simulink model "Tactical_SC_traincgf_4_15_Nov_27_Block"  (R2021a)
settings: Solver=VariableStepAuto  StartTime=0.0  StopTime=10.0  RelTol=1e-3
libraries: neural x66
(part 3 of 3)

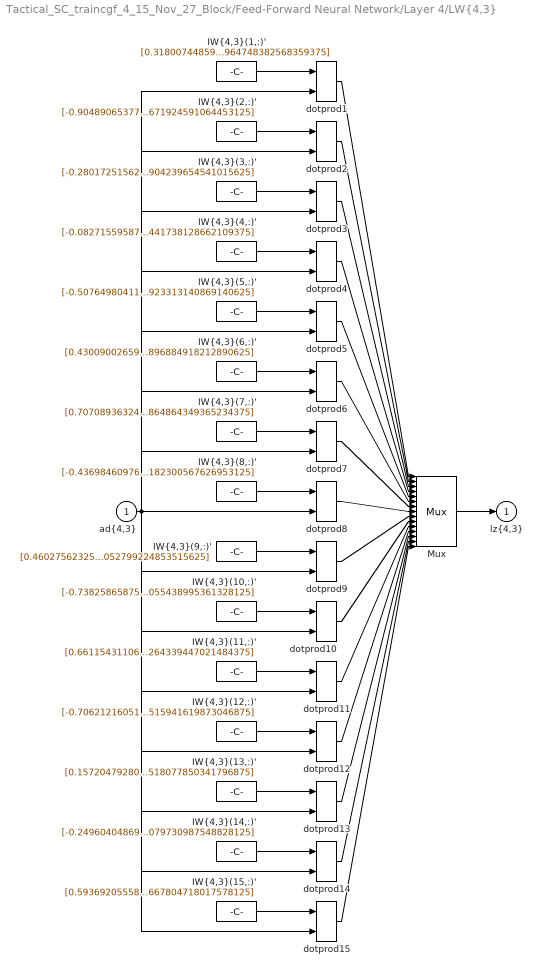
== system Tactical_SC_traincgf_4_15_Nov_27_Block/Feed-Forward Neural Network/Layer 4/LW{4,3} ==
  "ad{4,3}" : Inport  PortDimensions=15
      mask Display: e = 0.06;c1 = [120 230 180]/255;c2 = ([120 230 180]+0)/(256+128);c3 = ([120 230 180]+128)/(256+128);patch([0 1 1 0],[0 0 1 1],c1);patch([0 1 1 1-e 1-e 0+e],[0 0 1 1-e 0+e 0+e],c2);patch([0 0 1 1-e 0+e 0+e],[0 1 1 1-e 1-e 0+e],c3);plot([0 1 1 0 0],[0 0 1 1 0]);
  "IW{4,3}(1,:)'" : Constant  Value=[0.318007448593325692254296654937206767499446868896484375;0.0075615715523118520735579295433126389980316162109375;-0.96361569277834124847004204639233648777008056640625;0.860487806043781500164868702995590865612030029296875;0.7524752577316433654885940995882265269756317138671875;0.0077755469209772609673336773994378745555877685546875;-0.422356185153830387957185621417011134326457977294921875;0.6601121326122356691712411702610552310943603515625;0.510717921416298015202528404188342392444610595703125;-0.1037827559143178479672542380285449326038360595703125;-0.21994697437200461109796378877945244312286376953125;-0.7659263609886843848784110377891920506954193115234375;0.6680132640011307021410402740002609789371490478515625;0.99866317249397440480862542244722135365009307861328125;0.86246253723063259766234978087595663964748382568359375]
      mask Display: e = 0.06;c1 = [120 150 230]/255;c2 = ([120 150 230]+0)/383;c3 = ([120 150 230]+128)/383;patch([0 1 1 0],[0 0 1 1],c1);patch([0 1 1 1-e 1-e 0+e],[0 0 1 1-e 0+e 0+e],c2);patch([0 0 1 1-e 0+e 0+e],[0 1 1 1-e 1-e 0+e],c3);plot([0 1 1 0 0],[0 0 1 1 0]);disp('weights');
  "IW{4,3}(10,:)'" : Constant  Value=[-0.73825865875039620167541443152003921568393707275390625;0.334240600080149885542368792812339961528778076171875;-0.34759286482494566872247787614469416439533233642578125;-0.8904164201605351269819266235572285950183868408203125;0.6651335768264690084805579317617230117321014404296875;-0.732992280677375429576159149291925132274627685546875;-0.932434493180203549655971073661930859088897705078125;-0.85344556112142255788199918242753483355045318603515625;0.73189389910298052743797825314686633646488189697265625;-0.2192027742775237986183611837986973114311695098876953125;0.7688100905519898997653172045829705893993377685546875;-0.2037382409373282854403441888280212879180908203125;-0.803239734476193678602840009261853992938995361328125;-0.1369989655326274424762544867917313240468502044677734375;-0.59536079412170039848462010922958143055438995361328125]
      mask Display: e = 0.06;c1 = [120 150 230]/255;c2 = ([120 150 230]+0)/383;c3 = ([120 150 230]+128)/383;patch([0 1 1 0],[0 0 1 1],c1);patch([0 1 1 1-e 1-e 0+e],[0 0 1 1-e 0+e 0+e],c2);patch([0 0 1 1-e 0+e 0+e],[0 1 1 1-e 1-e 0+e],c3);plot([0 1 1 0 0],[0 0 1 1 0]);disp('weights');
  "IW{4,3}(11,:)'" : Constant  Value=[0.6611543110624340524594799717306159436702728271484375;0.172879229357835839664403465576469898223876953125;-0.73239400543458577086397554012364707887172698974609375;-0.388976697640453117355008316735620610415935516357421875;-0.1647486253821566493105166273380746133625507354736328125;-0.9568882255930060143356286062044091522693634033203125;-0.08967440119208837379094489961062208749353885650634765625;-0.1867190373629059318982825743660214357078075408935546875;0.74064277100053121927203392260707914829254150390625;-0.53590128485240129396771635583718307316303253173828125;0.4417113416338629416912908709491603076457977294921875;0.03073443842314471652343854657374322414398193359375;-0.67744238093146780244069304899312555789947509765625;0.69070075771987549106967207990237511694431304931640625;-0.090605605861847793303098796968697570264339447021484375]
      mask Display: e = 0.06;c1 = [120 150 230]/255;c2 = ([120 150 230]+0)/383;c3 = ([120 150 230]+128)/383;patch([0 1 1 0],[0 0 1 1],c1);patch([0 1 1 1-e 1-e 0+e],[0 0 1 1-e 0+e 0+e],c2);patch([0 0 1 1-e 0+e 0+e],[0 1 1 1-e 1-e 0+e],c3);plot([0 1 1 0 0],[0 0 1 1 0]);disp('weights');
  "IW{4,3}(12,:)'" : Constant  Value=[-0.7062121605125781798051320947706699371337890625;0.3502248328102306462739079506718553602695465087890625;-0.29514974520824022174991796418908052146434783935546875;-0.910971163136844896968113971524871885776519775390625;-0.04374406409938964845895981170542654581367969512939453125;0.11968141174501933932106112479232251644134521484375;0.264553137550485095719210448805824853479862213134765625;0.331907915136774145370424093925976194441318511962890625;0.126991008466725119330220650226692669093608856201171875;0.451463364557955715294923493274836800992488861083984375;-0.9627744505472277669611003148020245134830474853515625;0.315061084191821993982784988475032150745391845703125;0.2361511563990832396342511856346391141414642333984375;-0.2392189610648267628079111091210506856441497802734375;-0.146865284912714055831628456871840171515941619873046875]
      mask Display: e = 0.06;c1 = [120 150 230]/255;c2 = ([120 150 230]+0)/383;c3 = ([120 150 230]+128)/383;patch([0 1 1 0],[0 0 1 1],c1);patch([0 1 1 1-e 1-e 0+e],[0 0 1 1-e 0+e 0+e],c2);patch([0 0 1 1-e 0+e 0+e],[0 1 1 1-e 1-e 0+e],c3);plot([0 1 1 0 0],[0 0 1 1 0]);disp('weights');
  "IW{4,3}(13,:)'" : Constant  Value=[0.1572047928025288310305285222057136707007884979248046875;-0.2779559016106782909361072597675956785678863525390625;-0.7640312274407909942652850077138282358646392822265625;-0.604037151232293734182121625053696334362030029296875;0.1039704250373072458302203813218511641025543212890625;-0.3983619638610218505192506199819035828113555908203125;0.06345107524350544758728887018150999210774898529052734375;0.8674513190918593519285195725387893617153167724609375;0.166115950281934543486528355060727335512638092041015625;-0.46473978853246522557896014404832385480403900146484375;0.3495529342565715236190726500353775918483734130859375;0.9018303965299183655446313423453830182552337646484375;0.7396095696434386024264995285193435847759246826171875;0.27563280297923220540923239241237752139568328857421875;0.92522961385834878722533858308452181518077850341796875]
      mask Display: e = 0.06;c1 = [120 150 230]/255;c2 = ([120 150 230]+0)/383;c3 = ([120 150 230]+128)/383;patch([0 1 1 0],[0 0 1 1],c1);patch([0 1 1 1-e 1-e 0+e],[0 0 1 1-e 0+e 0+e],c2);patch([0 0 1 1-e 0+e 0+e],[0 1 1 1-e 1-e 0+e],c3);plot([0 1 1 0 0],[0 0 1 1 0]);disp('weights');
  "IW{4,3}(14,:)'" : Constant  Value=[-0.2496040486909129330062029339387663640081882476806640625;0.24055685414217098383460324839688837528228759765625;0.77732094229939596718992333990172483026981353759765625;0.436514146718682827241764243808574974536895751953125;-0.445911323119876523701776704911026172339916229248046875;0.878819427746916570498569853953085839748382568359375;-0.285655534964172563849871266938862390816211700439453125;0.620303798530214667295012986869551241397857666015625;-0.69046142052182946091676285504945553839206695556640625;0.81167656367563367769690785280545242130756378173828125;-0.1229823515269743428035553733934648334980010986328125;0.444697028654995829555218733730725944042205810546875;0.9206352224126470584764092564000748097896575927734375;0.60650102629068836090908689584466628730297088623046875;0.2377285168034162510242168764307280071079730987548828125]
      mask Display: e = 0.06;c1 = [120 150 230]/255;c2 = ([120 150 230]+0)/383;c3 = ([120 150 230]+128)/383;patch([0 1 1 0],[0 0 1 1],c1);patch([0 1 1 1-e 1-e 0+e],[0 0 1 1-e 0+e 0+e],c2);patch([0 0 1 1-e 0+e 0+e],[0 1 1 1-e 1-e 0+e],c3);plot([0 1 1 0 0],[0 0 1 1 0]);disp('weights');
  "IW{4,3}(15,:)'" : Constant  Value=[0.59369205558419835266903419324080459773540496826171875;0.6223017702005704254730744651169516146183013916015625;-0.82303653443154389801605930188088677823543548583984375;0.447647643950220885944446536086616106331348419189453125;0.478950635277783864918177414438105188310146331787109375;0.961807272093718079730706449481658637523651123046875;0.907417665800277717380595277063548564910888671875;-0.0279287499802652085245657787027084850706160068511962890625;0.78449887606904689096865013198112137615680694580078125;0.6276639944286017680497025139629840850830078125;-0.1243596416674599414164958943729288876056671142578125;-0.1998405092753248180059699734556488692760467529296875;0.173164233800528755136127756486530415713787078857421875;0.80725476240327120880380107337259687483310699462890625;0.394073676563273966877432030742056667804718017578125]
      mask Display: e = 0.06;c1 = [120 150 230]/255;c2 = ([120 150 230]+0)/383;c3 = ([120 150 230]+128)/383;patch([0 1 1 0],[0 0 1 1],c1);patch([0 1 1 1-e 1-e 0+e],[0 0 1 1-e 0+e 0+e],c2);patch([0 0 1 1-e 0+e 0+e],[0 1 1 1-e 1-e 0+e],c3);plot([0 1 1 0 0],[0 0 1 1 0]);disp('weights');
  "IW{4,3}(2,:)'" : Constant  Value=[-0.904890653772267850030175395659171044826507568359375;-0.0208113225532915446791548674809746444225311279296875;-0.8322529834342002885705369408242404460906982421875;-0.201960061930889001047262354404665529727935791015625;0.1648659289748206635550786813837476074695587158203125;0.293619332545560940417317397077567875385284423828125;0.601640573903069242334140653838403522968292236328125;0.698170959908910315760977027821354568004608154296875;-0.1659050925144660570964560974971391260623931884765625;-0.5886553210720730788807486533187329769134521484375;-0.004194114071626842132900492288172245025634765625;0.629363379037164438756235540495254099369049072265625;-0.7313233165425836457274044732912443578243255615234375;0.1070831469910651367882792328600771725177764892578125;-0.61843070398175559176934257266111671924591064453125]
      mask Display: e = 0.06;c1 = [120 150 230]/255;c2 = ([120 150 230]+0)/383;c3 = ([120 150 230]+128)/383;patch([0 1 1 0],[0 0 1 1],c1);patch([0 1 1 1-e 1-e 0+e],[0 0 1 1-e 0+e 0+e],c2);patch([0 0 1 1-e 0+e 0+e],[0 1 1 1-e 1-e 0+e],c3);plot([0 1 1 0 0],[0 0 1 1 0]);disp('weights');
  "IW{4,3}(3,:)'" : Constant  Value=[-0.2801725156256142934552144652116112411022186279296875;0.754097446770087831424689284176565706729888916015625;0.9614352930014380405054907896555960178375244140625;-0.89902945368803965919823895092122256755828857421875;-0.83854787826719501264705058929393999278545379638671875;-0.384508835938118576081024002633057534694671630859375;0.78776955048410834958616533185704611241817474365234375;-0.25780397740523997018868840314098633825778961181640625;0.984262714168782082424513646401464939117431640625;0.8275349590010059319666879673604853451251983642578125;0.389610385344987708577946250443346798419952392578125;-0.3502891227389819395199310747557319700717926025390625;-0.8684364926597070155622759557445533573627471923828125;0.040764357017907766611575226534114335663616657257080078125;-0.464077305096509518111957959263236261904239654541015625]
      mask Display: e = 0.06;c1 = [120 150 230]/255;c2 = ([120 150 230]+0)/383;c3 = ([120 150 230]+128)/383;patch([0 1 1 0],[0 0 1 1],c1);patch([0 1 1 1-e 1-e 0+e],[0 0 1 1-e 0+e 0+e],c2);patch([0 0 1 1-e 0+e 0+e],[0 1 1 1-e 1-e 0+e],c3);plot([0 1 1 0 0],[0 0 1 1 0]);disp('weights');
  "IW{4,3}(4,:)'" : Constant  Value=[-0.0827155958793168444298515851187403313815593719482421875;-0.2937163741220889523475534588214941322803497314453125;0.310757925464084483468951702889171428978443145751953125;-0.312646539431700676292535945322015322744846343994140625;0.85891004195614339966624584121746011078357696533203125;-0.7225507278437108826807389050372876226902008056640625;0.192825028394793596131506774327135644853115081787109375;0.1841770518927116351282080586315714754164218902587890625;1.004435028017355957530298837809823453426361083984375;0.542695336441261222404364161775447428226470947265625;0.6687380021998754475731630009249784052371978759765625;-0.507543771530717169326862858724780380725860595703125;-0.822728066329476259710418162285350263118743896484375;-0.329471420762690370143133122837753035128116607666015625;0.8070515688649171348600930286920629441738128662109375]
      mask Display: e = 0.06;c1 = [120 150 230]/255;c2 = ([120 150 230]+0)/383;c3 = ([120 150 230]+128)/383;patch([0 1 1 0],[0 0 1 1],c1);patch([0 1 1 1-e 1-e 0+e],[0 0 1 1-e 0+e 0+e],c2);patch([0 0 1 1-e 0+e 0+e],[0 1 1 1-e 1-e 0+e],c3);plot([0 1 1 0 0],[0 0 1 1 0]);disp('weights');
  "IW{4,3}(5,:)'" : Constant  Value=[-0.5076498041192991639292131367255933582782745361328125;-0.1011128868565034366611143923364579677581787109375;-0.531737091336316414214024916873313486576080322265625;0.469753227964551711703933278840850107371807098388671875;0.6103536927369519471398007226525805890560150146484375;-0.04885413240487412878110262681730091571807861328125;0.75028146985276100711104163565323688089847564697265625;0.74346871291821325922200003333273343741893768310546875;0.73432184803446765020140674096182920038700103759765625;0.775747382361128945404971091193147003650665283203125;0.2192593793514647781961457440047524869441986083984375;-0.31457355775344097992274328134953975677490234375;-0.68883644966301071921321863555931486189365386962890625;-0.157010608407656626628323692784761078655719757080078125;0.1845767123463361303326024653870263136923313140869140625]
      mask Display: e = 0.06;c1 = [120 150 230]/255;c2 = ([120 150 230]+0)/383;c3 = ([120 150 230]+128)/383;patch([0 1 1 0],[0 0 1 1],c1);patch([0 1 1 1-e 1-e 0+e],[0 0 1 1-e 0+e 0+e],c2);patch([0 0 1 1-e 0+e 0+e],[0 1 1 1-e 1-e 0+e],c3);plot([0 1 1 0 0],[0 0 1 1 0]);disp('weights');
  "IW{4,3}(6,:)'" : Constant  Value=[0.430090026592353069645469076931476593017578125;0.9270605736868537949391111396835185587406158447265625;-0.1930177137508202189764006106997840106487274169921875;0.59348617386316016020231245420291088521480560302734375;-0.4281062871592735685766228925785981118679046630859375;-0.2750814383625079795336887400480918586254119873046875;0.89083156503134330872484270003042183816432952880859375;0.86700321701421056985736868227832019329071044921875;-0.2151006258830908401957771047818823717534542083740234375;-0.4299160184834975861889461157261393964290618896484375;0.1494743217128160495121846906840801239013671875;-0.24861571998082343526448312331922352313995361328125;-0.339497802342841048517385615923558361828327178955078125;-0.009281429341859680215431893657296313904225826263427734375;0.01479249370185496161023142036583521985448896884918212890625]
      mask Display: e = 0.06;c1 = [120 150 230]/255;c2 = ([120 150 230]+0)/383;c3 = ([120 150 230]+128)/383;patch([0 1 1 0],[0 0 1 1],c1);patch([0 1 1 1-e 1-e 0+e],[0 0 1 1-e 0+e 0+e],c2);patch([0 0 1 1-e 0+e 0+e],[0 1 1 1-e 1-e 0+e],c3);plot([0 1 1 0 0],[0 0 1 1 0]);disp('weights');
  "IW{4,3}(7,:)'" : Constant  Value=[0.70708936324247384508367986200028099119663238525390625;-0.9154044041709143986196295372792519629001617431640625;-0.75151594573325775083816324695362709462642669677734375;0.0898117964893430098527460359036922454833984375;0.086933199946696071425122909204219467937946319580078125;0.5762268567970945110090497109922580420970916748046875;0.09406205343112995775900486705722869373857975006103515625;0.337592595210584545117882271370035596191883087158203125;-0.1045719515715654301946102577858255244791507720947265625;0.3355177246428036053060850463225506246089935302734375;-0.3479156581544173842956979569862596690654754638671875;0.093107586165917854970075495657511055469512939453125;-0.40797000697141638791975992717198096215724945068359375;-0.86789237710187372432102392849628813564777374267578125;0.2197605166413617305831706971730454824864864349365234375]
      mask Display: e = 0.06;c1 = [120 150 230]/255;c2 = ([120 150 230]+0)/383;c3 = ([120 150 230]+128)/383;patch([0 1 1 0],[0 0 1 1],c1);patch([0 1 1 1-e 1-e 0+e],[0 0 1 1-e 0+e 0+e],c2);patch([0 0 1 1-e 0+e 0+e],[0 1 1 1-e 1-e 0+e],c3);plot([0 1 1 0 0],[0 0 1 1 0]);disp('weights');
  "IW{4,3}(8,:)'" : Constant  Value=[-0.4369846097628933279111151932738721370697021484375;0.945916668281269412688061493099667131900787353515625;-0.462873560102180281461414779187180101871490478515625;0.371501187822665113191789032498490996658802032470703125;0.96988729620033009570789772624266333878040313720703125;0.5605916416882192887527480706921778619289398193359375;0.45657130501295617452939268332556821405887603759765625;-0.586437478571041115316120340139605104923248291015625;-0.51038786672779090647367183919413946568965911865234375;0.32274431627217070595037284874706529080867767333984375;-0.087150798296506071238809454371221363544464111328125;0.1238403085319534913111283458420075476169586181640625;-0.97643451727743535428771792794577777385711669921875;0.7751331730211836745780829005525447428226470947265625;0.6386921745650060433519001890090294182300567626953125]
      mask Display: e = 0.06;c1 = [120 150 230]/255;c2 = ([120 150 230]+0)/383;c3 = ([120 150 230]+128)/383;patch([0 1 1 0],[0 0 1 1],c1);patch([0 1 1 1-e 1-e 0+e],[0 0 1 1-e 0+e 0+e],c2);patch([0 0 1 1-e 0+e 0+e],[0 1 1 1-e 1-e 0+e],c3);plot([0 1 1 0 0],[0 0 1 1 0]);disp('weights');
  "IW{4,3}(9,:)'" : Constant  Value=[0.46027562325458293290836309097358025610446929931640625;-0.6215863137552479766867463695234619081020355224609375;-0.48180028837611599268342388313612900674343109130859375;0.78756321134661411154098686893121339380741119384765625;0.43159052574080047914861779645434580743312835693359375;0.33702442850708980159879502025432884693145751953125;0.1503460253569864069067563150383648462593555450439453125;0.31006894540027796214332056479179300367832183837890625;0.56138534642691995113494840552448295056819915771484375;-0.75864622309929730104016698533087037503719329833984375;0.4275911664662690458982297059264965355396270751953125;-0.20835554275199807960916587035171687602996826171875;0.07360618148284547856974313617683947086334228515625;-0.87628825689594214143340877853916026651859283447265625;0.06128309324566062754602313589202822186052799224853515625]
      mask Display: e = 0.06;c1 = [120 150 230]/255;c2 = ([120 150 230]+0)/383;c3 = ([120 150 230]+128)/383;patch([0 1 1 0],[0 0 1 1],c1);patch([0 1 1 1-e 1-e 0+e],[0 0 1 1-e 0+e 0+e],c2);patch([0 0 1 1-e 0+e 0+e],[0 1 1 1-e 1-e 0+e],c3);plot([0 1 1 0 0],[0 0 1 1 0]);disp('weights');
  Mux : Mux  Inputs=15
      mask Display: e = 0.06;c1 = [120 150 230]/255;c2 = ([120 150 230]+0)/383;c3 = ([120 150 230]+128)/383;patch([0 1 1 0],[0 0 1 1],c1);patch([0 1 1 1-e 1-e 0+e],[0 0 1 1-e 0+e 0+e],c2);patch([0 0 1 1-e 0+e 0+e],[0 1 1 1-e 1-e 0+e],c3);plot([0 1 1 0 0],[0 0 1 1 0]);disp('Mux');
  dotprod{1..15} (15 alike) : neural/Weight Functions/dotprod
  "lz{4,3}" : Outport
      mask Display: e = 0.06;c1 = [120 230 180]/255;c2 = ([120 230 180]+0)/(256+128);c3 = ([120 230 180]+128)/(256+128);patch([0 1 1 0],[0 0 1 1],c1);patch([0 1 1 1-e 1-e 0+e],[0 0 1 1-e 0+e 0+e],c2);patch([0 0 1 1-e 0+e 0+e],[0 1 1 1-e 1-e 0+e],c3);plot([0 1 1 0 0],[0 0 1 1 0]);
  wires:
  "IW{4,3}(1,:)'"/1 -> dotprod1/1
  "ad{4,3}"/1 -> dotprod1/2, dotprod2/2, dotprod3/2, dotprod4/2, dotprod5/2, dotprod6/2, dotprod7/2, dotprod8/2, dotprod9/2, dotprod10/2, dotprod11/2, dotprod12/2, dotprod13/2, dotprod14/2, dotprod15/2
  dotprod1/1 -> Mux/1
  "IW{4,3}(2,:)'"/1 -> dotprod2/1
  dotprod2/1 -> Mux/2
  "IW{4,3}(3,:)'"/1 -> dotprod3/1
  dotprod3/1 -> Mux/3
  "IW{4,3}(4,:)'"/1 -> dotprod4/1
  dotprod4/1 -> Mux/4
  "IW{4,3}(5,:)'"/1 -> dotprod5/1
  dotprod5/1 -> Mux/5
  "IW{4,3}(6,:)'"/1 -> dotprod6/1
  dotprod6/1 -> Mux/6
  "IW{4,3}(7,:)'"/1 -> dotprod7/1
  dotprod7/1 -> Mux/7
  "IW{4,3}(8,:)'"/1 -> dotprod8/1
  dotprod8/1 -> Mux/8
  "IW{4,3}(9,:)'"/1 -> dotprod9/1
  dotprod9/1 -> Mux/9
  "IW{4,3}(10,:)'"/1 -> dotprod10/1
  dotprod10/1 -> Mux/10
  "IW{4,3}(11,:)'"/1 -> dotprod11/1
  dotprod11/1 -> Mux/11
  "IW{4,3}(12,:)'"/1 -> dotprod12/1
  dotprod12/1 -> Mux/12
  "IW{4,3}(13,:)'"/1 -> dotprod13/1
  dotprod13/1 -> Mux/13
  "IW{4,3}(14,:)'"/1 -> dotprod14/1
  dotprod14/1 -> Mux/14
  "IW{4,3}(15,:)'"/1 -> dotprod15/1
  dotprod15/1 -> Mux/15
  Mux/1 -> "lz{4,3}"/1

== system Tactical_SC_traincgf_4_15_Nov_27_Block/Feed-Forward Neural Network/Layer 5/Delays 1 ==
  "p{5}" : Inport  PortDimensions=15
      mask Display: e = 0.06;c1 = [120 230 180]/255;c2 = ([120 230 180]+0)/(256+128);c3 = ([120 230 180]+128)/(256+128);patch([0 1 1 0],[0 0 1 1],c1);patch([0 1 1 1-e 1-e 0+e],[0 0 1 1-e 0+e 0+e],c2);patch([0 0 1 1-e 0+e 0+e],[0 1 1 1-e 1-e 0+e],c3);plot([0 1 1 0 0],[0 0 1 1 0]);
  mux : Mux  Inputs=1
      mask Display: e = 0.06;c1 = [120 150 230]/255;c2 = ([120 150 230]+0)/383;c3 = ([120 150 230]+128)/383;patch([0 1 1 0],[0 0 1 1],c1);patch([0 1 1 1-e 1-e 0+e],[0 0 1 1-e 0+e 0+e],c2);patch([0 0 1 1-e 0+e 0+e],[0 1 1 1-e 1-e 0+e],c3);plot([0 1 1 0 0],[0 0 1 1 0]);disp('Mux')
  "pd{5,4}" : Outport
      mask Display: e = 0.06;c1 = [120 230 180]/255;c2 = ([120 230 180]+0)/(256+128);c3 = ([120 230 180]+128)/(256+128);patch([0 1 1 0],[0 0 1 1],c1);patch([0 1 1 1-e 1-e 0+e],[0 0 1 1-e 0+e 0+e],c2);patch([0 0 1 1-e 0+e 0+e],[0 1 1 1-e 1-e 0+e],c3);plot([0 1 1 0 0],[0 0 1 1 0]);
  wires:
  "p{5}"/1 -> mux/1
  mux/1 -> "pd{5,4}"/1

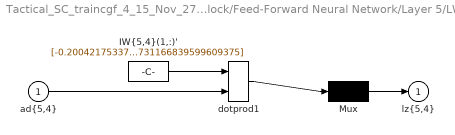
== system Tactical_SC_traincgf_4_15_Nov_27_Block/Feed-Forward Neural Network/Layer 5/LW{5,4} ==
  "ad{5,4}" : Inport  PortDimensions=15
      mask Display: e = 0.06;c1 = [120 230 180]/255;c2 = ([120 230 180]+0)/(256+128);c3 = ([120 230 180]+128)/(256+128);patch([0 1 1 0],[0 0 1 1],c1);patch([0 1 1 1-e 1-e 0+e],[0 0 1 1-e 0+e 0+e],c2);patch([0 0 1 1-e 0+e 0+e],[0 1 1 1-e 1-e 0+e],c3);plot([0 1 1 0 0],[0 0 1 1 0]);
  "IW{5,4}(1,:)'" : Constant  Value=[-0.20042175337175649474374949932098388671875;0.387505148267826893260235010529868304729461669921875;0.91392783733480154051420640826108865439891815185546875;0.64847881357920755807100476886262185871601104736328125;0.458415871290973442331306841879268176853656768798828125;-0.779630047288894179047247234848327934741973876953125;-0.2278505397525093789656835951973334886133670806884765625;0.176920348215999279073429306663456372916698455810546875;-0.07716941142593029823171235648260335437953472137451171875;-0.86633254978052198769233882558182813227176666259765625;-0.54069269902548489081794969024485908448696136474609375;0.6527227818278558135745015533757396042346954345703125;-0.98931297690328412475224695299402810633182525634765625;0.65019517438327401048780984638142399489879608154296875;-0.893967540675480787371043334132991731166839599609375]
      mask Display: e = 0.06;c1 = [120 150 230]/255;c2 = ([120 150 230]+0)/383;c3 = ([120 150 230]+128)/383;patch([0 1 1 0],[0 0 1 1],c1);patch([0 1 1 1-e 1-e 0+e],[0 0 1 1-e 0+e 0+e],c2);patch([0 0 1 1-e 0+e 0+e],[0 1 1 1-e 1-e 0+e],c3);plot([0 1 1 0 0],[0 0 1 1 0]);disp('weights');
  Mux : Mux  Inputs=1
      mask Display: e = 0.06;c1 = [120 150 230]/255;c2 = ([120 150 230]+0)/383;c3 = ([120 150 230]+128)/383;patch([0 1 1 0],[0 0 1 1],c1);patch([0 1 1 1-e 1-e 0+e],[0 0 1 1-e 0+e 0+e],c2);patch([0 0 1 1-e 0+e 0+e],[0 1 1 1-e 1-e 0+e],c3);plot([0 1 1 0 0],[0 0 1 1 0]);disp('Mux');
  dotprod1 : neural/Weight Functions/dotprod
  "lz{5,4}" : Outport
      mask Display: e = 0.06;c1 = [120 230 180]/255;c2 = ([120 230 180]+0)/(256+128);c3 = ([120 230 180]+128)/(256+128);patch([0 1 1 0],[0 0 1 1],c1);patch([0 1 1 1-e 1-e 0+e],[0 0 1 1-e 0+e 0+e],c2);patch([0 0 1 1-e 0+e 0+e],[0 1 1 1-e 1-e 0+e],c3);plot([0 1 1 0 0],[0 0 1 1 0]);
  wires:
  "IW{5,4}(1,:)'"/1 -> dotprod1/1
  "ad{5,4}"/1 -> dotprod1/2
  dotprod1/1 -> Mux/1
  Mux/1 -> "lz{5,4}"/1
